simulink model "modele_gyroBO1"  (Simulink 6.2)
settings: Solver=ode45  StartTime=0.0  StopTime=10.0  RelTol=1e-3
undefined symbols (not defined in the file or in its folder): K1, K2, K3, K4, Kamp, Km1, Km2, sigbuilder_block
libraries: library_gyro x2
settings Model: Creator=ahmed.chaibet  LastModifiedBy=Etudiant
settings HardwareCC: TargetUnknown=on

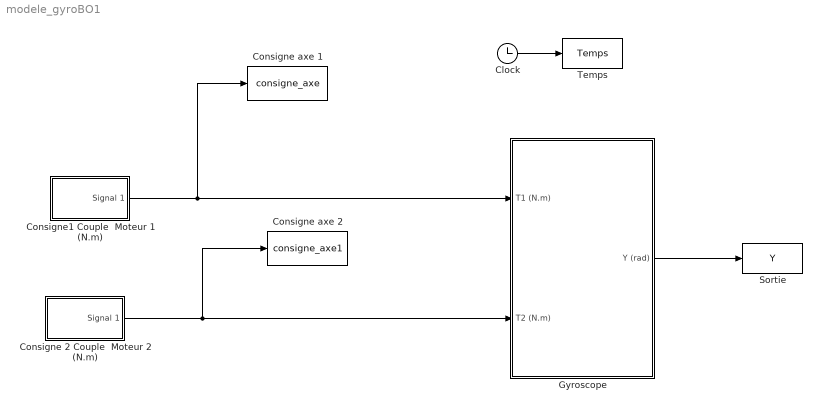
== system modele_gyroBO1 ==
  Clock : Clock
      settings: Decimation=10
  Consigne 2 Couple  Moteur 2 (N.m) : Subsystem  Tag=STV Subsys  LoadFcn=sigbuilder_block('load');  StartFcn=sigbuilder_block('start');  StopFcn=sigbuilder_block('stop');  ClipboardFcn=sigbuilder_block('clipboard');  mask(Sigbuilder block){}
      mask help: Sigbuilder GUI
      mask init:
      | if ~strcmp(get_param(bdroot(gcbh),'SimulationStatus'),'stopped') tuvar = sigbuilder_block('maskInit'); end
      settings: CopyFcn=sigbuilder_block('copy');  DeleteFcn=sigbuilder_block('delete');  ModelCloseFcn=sigbuilder_block('modelClose');  PreSaveFcn=sigbuilder_block('preSave');  NameChangeFcn=sigbuilder_block('namechange');  OpenFcn=sigbuilder_block('open',[204 195.75 550.5 399.75 ]);  CloseFcn=sigbuilder_block('close');
      mask Display: plot(0,0,100,100,[10,10,40,40,10],[80,20,20,80,80],[40,10],[50,50], [40,27,10],[65,72,56],[40,25,25,10],[28,28,43,43]);
  Consigne axe 1 : ToWorkspace  VariableName=consigne_axe  SampleTime=-1  SaveFormat=Array
  Consigne axe 2 : ToWorkspace  VariableName=consigne_axe1  SampleTime=-1  SaveFormat=Array
  Consigne1 Couple  Moteur 1 (N.m) : Subsystem  Tag=STV Subsys  LoadFcn=sigbuilder_block('load');  StartFcn=sigbuilder_block('start');  StopFcn=sigbuilder_block('stop');  ClipboardFcn=sigbuilder_block('clipboard');  mask(Sigbuilder block){}
      mask help: Sigbuilder GUI
      mask init:
      | if ~strcmp(get_param(bdroot(gcbh),'SimulationStatus'),'stopped') tuvar = sigbuilder_block('maskInit'); end
      settings: CopyFcn=sigbuilder_block('copy');  DeleteFcn=sigbuilder_block('delete');  ModelCloseFcn=sigbuilder_block('modelClose');  PreSaveFcn=sigbuilder_block('preSave');  NameChangeFcn=sigbuilder_block('namechange');  OpenFcn=sigbuilder_block('open',[204 195.75 550.5 399.75 ]);  CloseFcn=sigbuilder_block('close');
      mask Display: plot(0,0,100,100,[10,10,40,40,10],[80,20,20,80,80],[40,10],[50,50], [40,27,10],[65,72,56],[40,25,25,10],[28,28,43,43]);
  Gyroscope : Subsystem
  Sortie : ToWorkspace  VariableName=Y  SampleTime=-1  SaveFormat=Array
  Temps : ToWorkspace  VariableName=Temps  SampleTime=-1  SaveFormat=Array
  wires:
  Gyroscope/1(Y (rad)) -> Sortie/1
  Consigne1 Couple  Moteur 1 (N.m)/1(Signal 1) -> Gyroscope/1(T1 (N.m)), Consigne axe 1/1
  Consigne 2 Couple  Moteur 2 (N.m)/1(Signal 1) -> Gyroscope/2(T2 (N.m)), Consigne axe 2/1
  Clock/1 -> Temps/1

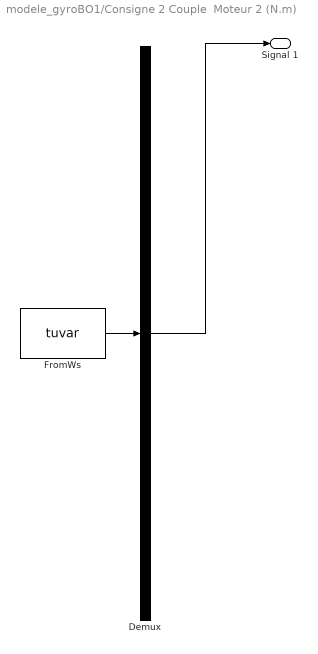
== system modele_gyroBO1/Consigne 2 Couple  Moteur 2 (N.m) ==
  Demux : Demux  Tag=STV Demux  Outputs=1
  FromWs : FromWorkspace  Tag=STV FromWs  VariableName=tuvar  SampleTime=0  SigBuilderData=DataTag0
      SigBuilderData=|
      | channels.xData = [0 1 1 3]
      | channels.yData = [0 0 -1 -0.995]
      | channels.label = 'Signal 1'
      | common.afterFinalStr = 'Extrapolate'
      | common.sampleTime = 0
      | dataSet.timeRange = [0 3]
      | dataSet.name = 'Group 1'
  Signal 1 : Outport  Tag=STV Outport
  wires:
  FromWs/1 -> Demux/1
  Demux/1 -> Signal 1/1

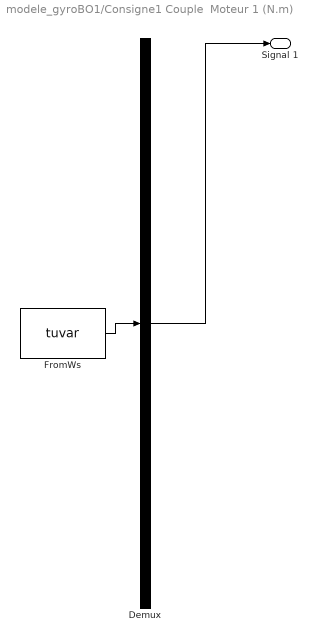
== system modele_gyroBO1/Consigne1 Couple  Moteur 1 (N.m) ==
  Demux : Demux  Tag=STV Demux  Outputs=1
  FromWs : FromWorkspace  Tag=STV FromWs  VariableName=tuvar  SampleTime=0  SigBuilderData=DataTag1
      SigBuilderData=|
      | channels.xData = [0 1 1 3.02 3.02 10]
      | channels.yData = [0 0 1 1 0 0]
      | channels.label = 'Signal 1'
      | common.afterFinalStr = 'Extrapolate'
      | common.sampleTime = 0
      | dataSet.timeRange = [0 10]
      | dataSet.name = 'Group 1'
  Signal 1 : Outport  Tag=STV Outport
  wires:
  Demux/1 -> Signal 1/1
  FromWs/1 -> Demux/1

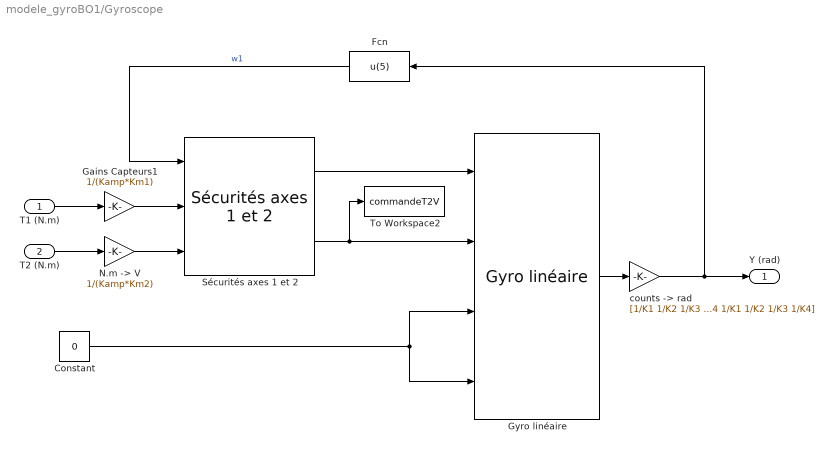
== system modele_gyroBO1/Gyroscope ==
  T1 (N.m) : Inport  Port=1  OutDataType=fixdt(1,16,0)  OutScaling=[]  LatchInput=off
  T2 (N.m) : Inport  Port=2  OutDataType=fixdt(1,16,0)  OutScaling=[]  LatchInput=off
  Constant : Constant  Value=0  OutDataType=fixdt(1,16,0)  OutScaling=[]
  Fcn : Fcn  Orientation=left  Expr=u(5)
  Gains Capteurs1 : Gain  Gain=1/(Kamp*Km1)  ParameterDataType=fixdt(1,16,0)  ParameterScaling=[]  OutDataType=fixdt(1,16,0)  OutScaling=[]  SaturateOnIntegerOverflow=on
  Gyro linéaire : library_gyro/Gyro linéaire
  "N.m -> V" : Gain  Gain=1/(Kamp*Km2)  ParameterDataType=fixdt(1,16,0)  ParameterScaling=[]  OutDataType=fixdt(1,16,0)  OutScaling=[]  SaturateOnIntegerOverflow=on
  Sécurités axes 1 et 2 : library_gyro/Sécurités axes 1 et 2
  To Workspace2 : ToWorkspace  VariableName=commandeT2V  SampleTime=-1  SaveFormat=Array
  "counts -> rad" : Gain  Gain=[1/K1 1/K2 1/K3 1/K4 1/K1 1/K2 1/K3 1/K4]  ParameterDataType=fixdt(1,16,0)  ParameterScaling=[]  OutDataType=fixdt(1,16,0)  OutScaling=[]  SaturateOnIntegerOverflow=on
  Y (rad) : Outport
  wires:
  Sécurités axes 1 et 2/2 -> Gyro linéaire/2, To Workspace2/1
  Sécurités axes 1 et 2/1 -> Gyro linéaire/1
  Gyro linéaire/1 -> "counts -> rad"/1
  "counts -> rad"/1 -> Y (rad)/1, Fcn/1
  T1 (N.m)/1 -> Gains Capteurs1/1
  T2 (N.m)/1 -> "N.m -> V"/1
  Gains Capteurs1/1 -> Sécurités axes 1 et 2/2
  "N.m -> V"/1 -> Sécurités axes 1 et 2/3
  Constant/1 -> Gyro linéaire/3, Gyro linéaire/4
  Fcn/1 -> Sécurités axes 1 et 2/1  "w1"
